simulink model "sistemacompensado"  (R2020b)
settings: Solver=VariableStepAuto  StartTime=0.0  StopTime=60.0  RelTol=1e-3
settings Model: Creator=Advance  LastModifiedBy=Advance

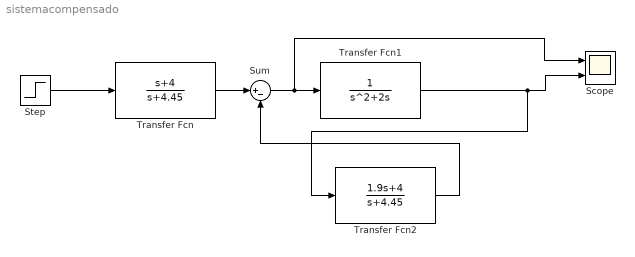
== system sistemacompensado ==
  Scope : Scope  NumInputPorts=2
  Step : Step  Time=0  After=100  SampleTime=0
  Sum : Sum  Inputs=|+-
  Transfer Fcn : TransferFcn  Numerator=[1 4]  Denominator=[1 4.45]
  Transfer Fcn1 : TransferFcn  Denominator=[1 2 0]
  Transfer Fcn2 : TransferFcn  Numerator="[1.9  4]"  Denominator=[1 4.45]
  wires:
  Step/1 -> Transfer Fcn/1
  Transfer Fcn/1 -> Sum/1
  Sum/1 -> Scope/1, Transfer Fcn1/1
  Transfer Fcn1/1 -> Transfer Fcn2/1, Scope/2
  Transfer Fcn2/1 -> Sum/2
